simulink subsystem "DCGearbox_SubSystem"  (R2020b)
settings: Solver=VariableStepAuto  StartTime=0.0  StopTime=10.0  RelTol=1e-3
values from neighbouring files (symbols this model uses):
  Beq = BeqEst    [loadParNominal.m]
  Jeq = mot.J+(mld.J/gbox.N1^2)    [loadParNominal.m]
undefined symbols (not defined in the file or in its folder): gbox, mld, mot, rads2rpm, sens
settings Model: Creator=umberto  LastModifiedBy=umbe

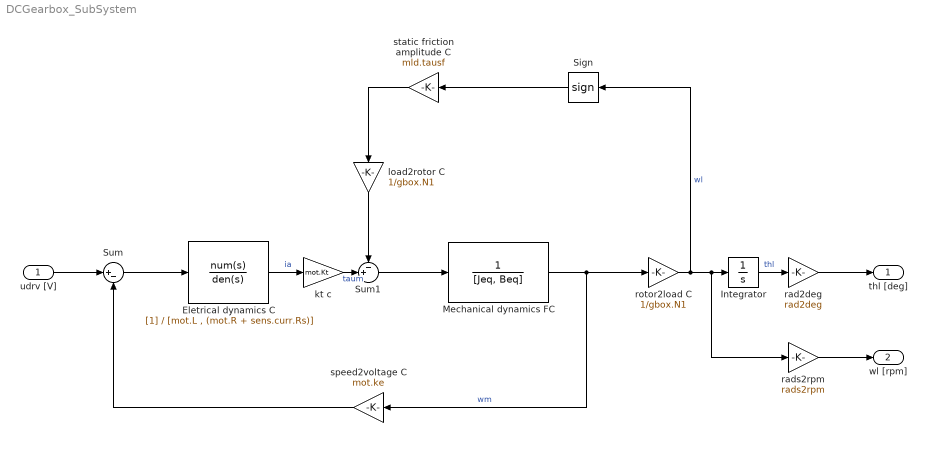
== system DCGearbox_SubSystem ==
  udrv [V] : Inport
  Eletrical dynamics C : TransferFcn  Denominator=[mot.L , (mot.R + sens.curr.Rs)]
  Integrator : Integrator
  Mechanical dynamics FC : TransferFcn  Denominator=[Jeq, Beq]
  Sign : Signum  ZeroCross=off
  Sum : Sum  Inputs=|+-
  Sum1 : Sum  Inputs=-+|
  kt c : Gain  Gain=mot.Kt
  load2rotor C : Gain  Gain=1/gbox.N1
  rad2deg : Gain  Gain=rad2deg
  rads2rpm : Gain  Gain=rads2rpm
  rotor2load C : Gain  Gain=1/gbox.N1
  speed2voltage C : Gain  Gain=mot.ke
  static friction amplitude C : Gain  Gain=mld.tausf
  thl [deg] : Outport
  wl [rpm] : Outport  Port=2
  wires:
  Sum/1 -> Eletrical dynamics C/1
  udrv [V]/1 -> Sum/1
  Eletrical dynamics C/1 -> kt c/1  "ia"
  kt c/1 -> Sum1/2  "taum"
  Sum1/1 -> Mechanical dynamics FC/1
  Mechanical dynamics FC/1 -> rotor2load C/1, speed2voltage C/1  "wm"
  speed2voltage C/1 -> Sum/2
  rotor2load C/1 -> rads2rpm/1, Integrator/1, Sign/1  "wl"
  Integrator/1 -> rad2deg/1  "thl"
  rads2rpm/1 -> wl [rpm]/1
  rad2deg/1 -> thl [deg]/1
  load2rotor C/1 -> Sum1/1
  static friction amplitude C/1 -> load2rotor C/1
  Sign/1 -> static friction amplitude C/1
